simulink model "inductor_skineffect"  (R2016b)
settings: Solver=ode45  StartTime=0.0  StopTime=tmax  FixedStep=dt  MaxStep=dt  RelTol=1e-4
values from neighbouring files (symbols this model uses):
  Afe = (do-di)/2*h    (= 8.75e-05)    [run_inductor.m]    (also in run_inductor_sweep.m)
  am = 0.5    [run_inductor.m]    (also in run_inductor_sweep.m)
  B0 = -1    [run_inductor.m]    (also in run_inductor_sweep.m)
  C = sigma*d^2*C    [run_inductor.m]    (also in run_inductor_sweep.m)
  cex = 0.3137    [run_inductor.m]    (also in run_inductor_sweep.m)
  Cinv = inv(C(2:end,2:end))    [run_inductor.m]    (also in run_inductor_sweep.m)
  delta = 0    [run_inductor.m]    (also in run_inductor_sweep.m)
  dens = 7650    [run_inductor.m]    (also in run_inductor_sweep.m)
  dt = deadtime/2    (= 5e-08)    [run_inductor.m]    (also in run_inductor_sweep.m = 0)
  f = 400    [run_inductor.m]    (also in run_inductor_sweep.m)
  lfe = (do+di)/2*pi    (= 0.359712358836)    [run_inductor.m]    (also in run_inductor_sweep.m)
  Lsig = 1.8735e-06    [run_inductor.m]    (also in run_inductor_sweep.m)
  N1 = 254    [run_inductor.m]    (also in run_inductor_sweep.m)
  nb = 1    [run_inductor.m]    (also in run_inductor_sweep.m)
  nu0 = 1/mu0    (= 795774.715459)    [run_inductor.m]    (also in run_inductor_sweep.m)
  R = 0.56    [run_inductor.m]    (also in run_inductor_sweep.m)
  Rfe = N1^2*Afe/lfe/(sigma*d^2/12-C(1,2:end)*Cinv*C(2:end,1))    [run_inductor.m]    (also in run_inductor_sweep.m)
  Udc = 128.11    [run_inductor.m]    (also in run_inductor_sweep.m)
  uphase = 0    [run_inductor.m]    (also in run_inductor_sweep.m)
  w = w/sum(w)    [run_inductor.m]    (also in run_inductor_sweep.m)
undefined symbols (not defined in the file or in its folder): alfa
libraries: powerlib x12, powerlib_meascontrol x6
settings Model: Creator=rasilo  LastModifiedBy=rasilo
settings SolverCC: ZeroCrossAlgorithm=Adaptive

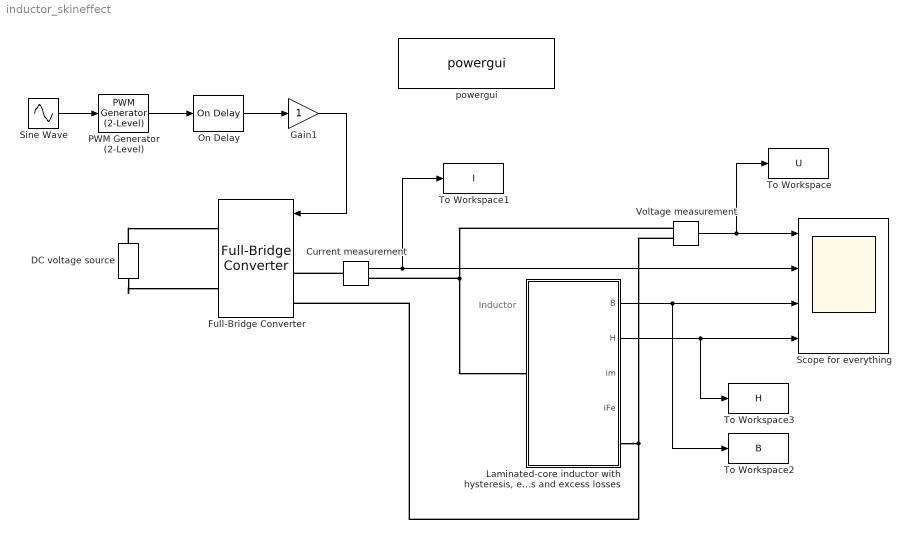
== system inductor_skineffect ==
  note: Inductor
  Current measurement : powerlib/Measurements/Current Measurement  PhasorSimulation=off  OutputType=Complex  PSBequivalent=0
  DC voltage source : powerlib/Electrical Sources/DC Voltage Source  Amplitude=Udc  Measurements=None
  Full-Bridge Converter : powerlib/Power Electronics/Full-Bridge Converter  ModelType=Switching devices  Ron=55e-3  Rs=1e6  Cs=1e-6  Vforward=[0,0]  Ron_Diode=1e-3  Rs_Diode=1e6  Cs_Diode=inf  Vf_Diode=1e-3  Rs_CurrentSource=inf
  Gain1 : Gain
  "Laminated-core inductor with hysteresis, eddy currents and excess losses" : Subsystem
  On Delay : powerlib_meascontrol/Logic/On Delay  DelayType=On delay  delay=deadtime  ic=0  Ts=0
  PWM Generator (2-Level) : powerlib_meascontrol/Pulse & Signal Generators/PWM Generator (2-Level)  ModulatorType=Single-phase full-bridge (4 pulses)  ModulatorMode=Unsynchronized  Fc=fcar  Pc=0  nF=27  MinMax="[ -1  1 ]"  SamplingTechnique=Natural  ModulatingSignals=off  m=0.8  Freq=60  Phase=0  Ts=0  ShowCarrierOutport=off
  Scope for everything : Scope  NumInputPorts=4
  Sine Wave : Sin  Amplitude=am  Frequency=2*pi*f  Phase=uphase  SampleTime=0
  To Workspace : ToWorkspace  VariableName=U  SaveFormat=Structure With Time  SampleTime=-1
  To Workspace1 : ToWorkspace  VariableName=I  SaveFormat=Structure With Time  SampleTime=-1
  To Workspace2 : ToWorkspace  VariableName=B  SampleTime=-1
  To Workspace3 : ToWorkspace  VariableName=H  SampleTime=-1
  Voltage measurement : powerlib/Measurements/Voltage Measurement  PhasorSimulation=off  OutputType=Complex  PSBequivalent=0
  powergui : powerlib/powergui  Priority=1  SimulationMode=Discrete  SolverType=Backward Euler  SampleTime=dt  frequency=60  SPID=off  DisableSnubberDevices=off  DisableRonSwitches=off  DisableVfSwitches=on  SwTol=0  DisplayEquations=on  Interpol=off  ExternalGateDelay=off  methode=off  Ts=0  FunctionMessages=off  echomessages=off  HookPort=off  EnableUseOfTLC=off  x0status=blocks  frequencyindice=0  Pbase=100e6  ErrMax=1e-4  Iterations=50  UnitsV=kV  UnitsW=MW  buscounter=0  RestoreLinks=warning  ResistiveCurrentMeasurement=off  Frange=[0:2:500]  Ylog=off  Xlog=on  ShowGrid=off  save=off  variable=ZData  structure=phase_a  ZoomFFT=off  StartTime=0.12  cycles=1  DisplayStyle=2  fundamental=50  FreqAxis=off  MaxFrequency=1000  frequencyindicesteady=1  RmsSteady=1  display=off
  wires:
  Voltage measurement/1 -> To Workspace/1, Scope for everything/1
  "Laminated-core inductor with hysteresis, eddy currents and excess losses"/2(H) -> To Workspace3/1, Scope for everything/4
  "Laminated-core inductor with hysteresis, eddy currents and excess losses"/1(B) -> To Workspace2/1, Scope for everything/3
  On Delay/1 -> Gain1/1
  Gain1/1 -> Full-Bridge Converter/1
  PWM Generator (2-Level)/1 -> On Delay/1
  Current measurement/1 -> To Workspace1/1, Scope for everything/2
  Sine Wave/1 -> PWM Generator (2-Level)/1
  connections:
  Voltage measurement/LConn2 -- Full-Bridge Converter/LConn2 -- "Laminated-core inductor with hysteresis, eddy currents and excess losses"/RConn1
  Current measurement/LConn1 -- Full-Bridge Converter/LConn1
  Voltage measurement/LConn1 -- "Laminated-core inductor with hysteresis, eddy currents and excess losses"/LConn1 -- Current measurement/RConn1
  DC voltage source/LConn1 -- Full-Bridge Converter/RConn2
  DC voltage source/RConn1 -- Full-Bridge Converter/RConn1

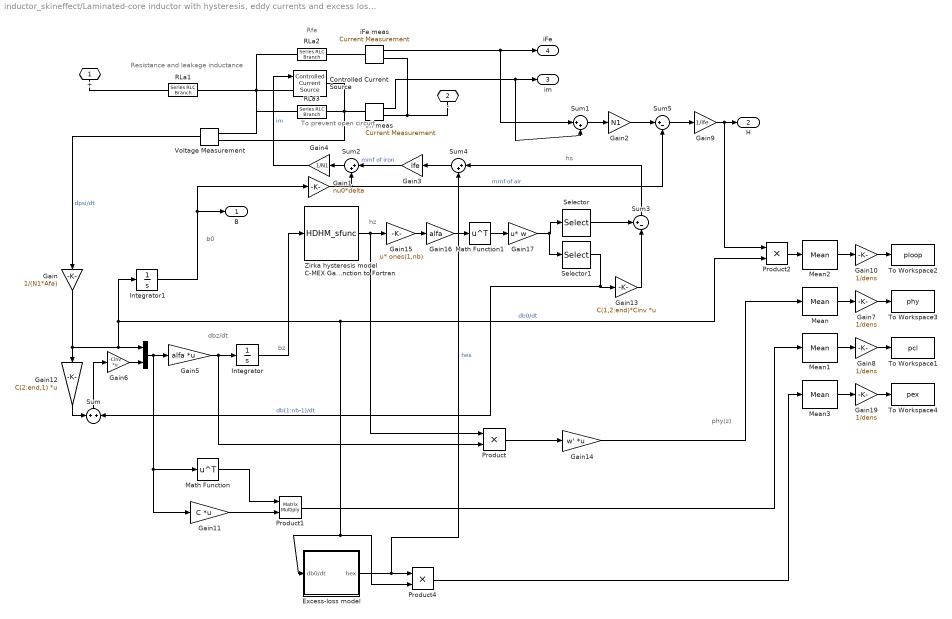
== system inductor_skineffect/Laminated-core inductor with hysteresis, eddy currents and excess losses ==
  note: phy(z)
  note: hs
  note: bz
  note: b0
  note: hz
  note: dbz/dt
  note: To prevent
      | open circuit
  note: Rfe
  note: Resistance and leakage inductance
  " " : Concatenate
  Controlled Current Source : powerlib/Electrical Sources/Controlled Current Source  Initialize=off  Source_Type=AC  Amplitude=0  Phase=0  Frequency=0  Measurements=None
  Excess-loss model : Subsystem
  Gain : Gain  Gain=1/(N1*Afe)
  Gain1 : Gain  Gain=nu0*delta
  Gain{7..8,10,19} (4 alike) : Gain  Gain=1/dens
  Gain11 : Gain  Gain=C  Multiplication=Matrix(K*u) (u vector)
  Gain12 : Gain  Gain=C(2:end,1)  Multiplication=Matrix(K*u) (u vector)
  Gain13 : Gain  Gain=C(1,2:end)*Cinv  Multiplication=Matrix(K*u) (u vector)
  Gain14 : Gain  Gain=w'  Multiplication=Matrix(K*u) (u vector)
  Gain15 : Gain  Gain=ones(1,nb)  Multiplication=Matrix(u*K)
  Gain16 : Gain  Gain=alfa
  Gain17 : Gain  Gain=w  Multiplication=Matrix(u*K)
  Gain2 : Gain  Gain=N1
  Gain3 : Gain  Gain=lfe
  Gain4 : Gain  Gain=1/N1
  Gain5 : Gain  Gain=alfa  Multiplication=Matrix(K*u) (u vector)
  Gain6 : Gain  Gain=-Cinv  Multiplication=Matrix(K*u) (u vector)
  Gain9 : Gain  Gain=1/lfe
  Integrator : Integrator  InitialCondition=B0
  Integrator1 : Integrator  InitialCondition=B0
  Math Function : Math  Operator=transpose  SaturateOnIntegerOverflow=on
  Math Function1 : Math  Operator=transpose  SaturateOnIntegerOverflow=on
  Mean{,1..3} (4 alike) : powerlib_meascontrol/Measurements/Mean  Freq=f  Vinit=0  Ts=0
  Product : Product
  Product1 : Product  Multiplication=Matrix(*)
  Product2 : Product
  Product4 : Product
  RLa1 : powerlib/Elements/Series RLC Branch  LConnTagsString=__new0  RConnTagsString=__new0  BranchType=RL  Resistance=R  Inductance=Lsig  SetiL0=off  InitialCurrent=0  Capacitance=1e-6  Setx0=off  InitialVoltage=0  Measurements=None
  RLa2 : powerlib/Elements/Series RLC Branch  LConnTagsString=__new0  RConnTagsString=__new0  BranchType=R  Resistance=Rfe  Inductance=1e-3  SetiL0=off  InitialCurrent=0  Capacitance=1e-6  Setx0=off  InitialVoltage=0  Measurements=None
  RLa3 : powerlib/Elements/Series RLC Branch  LConnTagsString=__new0  RConnTagsString=__new0  BranchType=R  Resistance=100e3  Inductance=1e-3  SetiL0=off  InitialCurrent=0  Capacitance=1e-6  Setx0=off  InitialVoltage=0  Measurements=None
  Selector : Selector  InputPortWidth=nb  IndexOptions=Index vector (dialog)  Indices=1  OutputSizes=1
  Selector1 : Selector  InputPortWidth=nb  IndexOptions=Index vector (dialog)  Indices=2:nb  OutputSizes=1
  Sum : Sum  Inputs=+|+
  Sum1 : Sum  Inputs=|++
  Sum2 : Sum  Inputs=|++
  Sum3 : Sum  Inputs=+-|
  Sum4 : Sum  Inputs=|++
  Sum5 : Sum  Inputs=|+-
  To Workspace1 : ToWorkspace  VariableName=pcl  SampleTime=-1
  To Workspace2 : ToWorkspace  VariableName=ploop  SampleTime=-1
  To Workspace3 : ToWorkspace  VariableName=phy  SampleTime=-1
  To Workspace4 : ToWorkspace  VariableName=pex  SampleTime=-1
  Voltage Measurement : powerlib/Measurements/Voltage Measurement  PhasorSimulation=off  OutputType=Complex  PSBequivalent=0
  Zirka hysteresis model C-MEX Gateway S-Function to Fortran : S-Function  FunctionName=HDHM_sfunc  Parameters=flag_hy  SFunctionDeploymentMode=off  EnableBusSupport=off
  iFe meas : powerlib/Measurements/Current Measurement  PhasorSimulation=off  OutputType=Complex  PSBequivalent=0
  im meas : powerlib/Measurements/Current Measurement  PhasorSimulation=off  OutputType=Complex  PSBequivalent=0
  + : PMIOPort  Port=1  Side=Left
  - : PMIOPort  Port=2  Side=Right
  B : Outport
  H : Outport  Port=2
  im : Outport  Port=3
  iFe : Outport  Port=4
  wires:
  Voltage Measurement/1 -> Gain/1  "dpsi/dt"
  Zirka hysteresis model C-MEX Gateway S-Function to Fortran/1 -> Product/1, Gain15/1
  Gain4/1 -> Controlled Current Source/1  "im"
  Gain3/1 -> Sum2/1  "mmf of iron"
  Sum2/1 -> Gain4/1
  Gain14/1 -> Mean/1
  Product1/1 -> Mean1/1
  Mean/1 -> Gain7/1
  Mean1/1 -> Gain8/1
  Gain7/1 -> To Workspace3/1
  Gain8/1 -> To Workspace1/1
  Integrator/1 -> Zirka hysteresis model C-MEX Gateway S-Function to Fortran/1
  " "/1 -> Math Function/1, Gain11/1, Gain5/1
  Integrator1/1 -> Gain1/1, B/1
  Selector/1 -> Sum3/1
  Gain5/1 -> Product/2, Integrator/1
  Product/1 -> Gain14/1
  Math Function/1 -> Product1/1
  Gain11/1 -> Product1/2
  Gain1/1 -> Sum5/2, Sum2/2  "mmf of air"
  iFe meas/1 -> iFe/1, Sum1/1
  im meas/1 -> Sum1/2, im/1
  Sum1/1 -> Gain2/1
  Gain2/1 -> Sum5/1
  Sum5/1 -> Gain9/1
  Selector1/1 -> Sum/2, Gain13/1  "db(1:nb-1)/dt"
  Gain13/1 -> Sum3/2
  Gain6/1 -> " "/2
  Gain12/1 -> Sum/1
  Sum/1 -> Gain6/1
  Product2/1 -> Mean2/1
  Gain9/1 -> Product2/1, H/1
  Mean2/1 -> Gain10/1
  Gain10/1 -> To Workspace2/1
  Gain15/1 -> Gain16/1
  Gain16/1 -> Math Function1/1
  Math Function1/1 -> Gain17/1
  Gain17/1 -> Selector1/1, Selector/1
  Gain/1 -> " "/1, Integrator1/1, Excess-loss model/1(db0/dt), Product4/2, Product2/2, Gain12/1  "db0/dt"
  Mean3/1 -> Gain19/1
  Gain19/1 -> To Workspace4/1
  Product4/1 -> Mean3/1
  Sum4/1 -> Gain3/1
  Sum3/1 -> Sum4/1
  Excess-loss model/1(hex) -> Sum4/2, Product4/1  "hex"
  connections:
  im meas/RConn1 -- iFe meas/RConn1 -- -/RConn1
  RLa1/RConn1 -- RLa2/LConn1 -- Voltage Measurement/LConn1 -- RLa3/LConn1 -- Controlled Current Source/LConn1
  +/RConn1 -- RLa1/LConn1
  Voltage Measurement/LConn2 -- Controlled Current Source/RConn1 -- im meas/LConn1 -- RLa3/RConn1
  RLa2/RConn1 -- iFe meas/LConn1

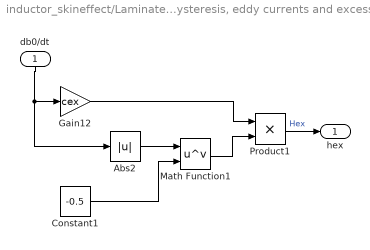
== system inductor_skineffect/Laminated-core inductor with hysteresis, eddy currents and excess losses/Excess-loss model ==
  db0/dt : Inport
  Abs2 : Abs
  Constant1 : Constant  Value=-0.5
  Gain12 : Gain  Gain=cex
  Math Function1 : Math  Operator=pow  SaturateOnIntegerOverflow=on
  Product1 : Product
  hex : Outport
  wires:
  Constant1/1 -> Math Function1/2
  Abs2/1 -> Math Function1/1
  Math Function1/1 -> Product1/2
  Gain12/1 -> Product1/1
  Product1/1 -> hex/1  "Hex"
  db0/dt/1 -> Gain12/1, Abs2/1
